simulink model "closedloop_voltage_simulation_1999v"  (R2023a)
settings: Solver=ode45  StartTime=0.0  StopTime=0.3  MaxStep=1e-4  RelTol=1e-3
settings Model: Creator=angie  LastModifiedBy=angie

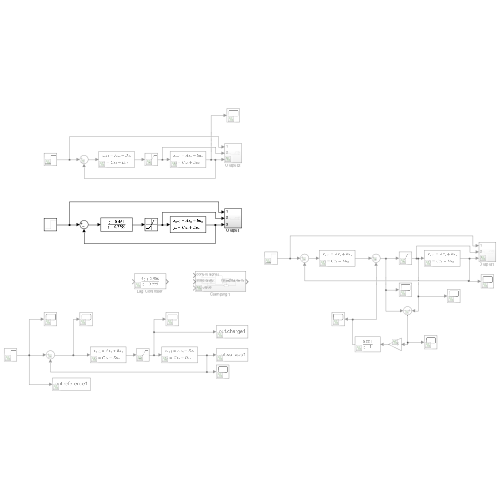
[thumbnail: Simulink's stored preview of the top-level diagram]
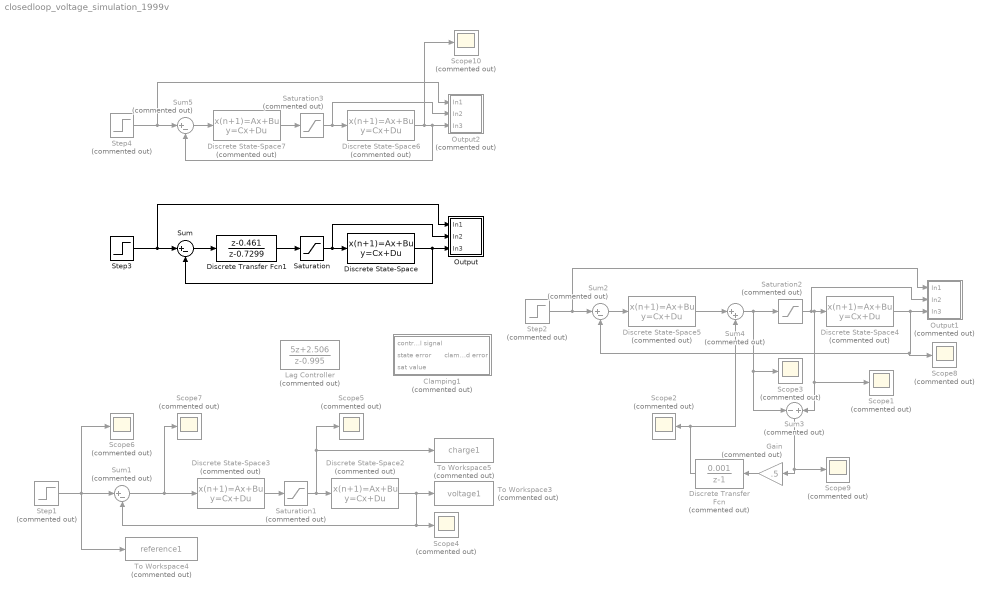
== system closedloop_voltage_simulation_1999v ==
  Clamping1 : Subsystem  Commented=on
  Discrete Transfer Fcn : DiscreteTransferFcn  Commented=on  Numerator=[0.001]  Denominator=[1 -1]  SampleTime=0.001
  Discrete Transfer Fcn1 : DiscreteTransferFcn  Numerator=[1, -0.461]  Denominator=[1 -0.7299]  SampleTime=0.001
  Discrete State-Space : DiscreteStateSpace  B=0.2728  D=0  InitialCondition=0/6  SampleTime=1/1000
  Discrete State-Space2 : DiscreteStateSpace  Commented=on  B=0.01185  D=0  InitialCondition=2000/6000  SampleTime=1/2000
  Discrete State-Space3 : DiscreteStateSpace  Commented=on  A=0.961  B=0.5099  C=0.826  D=5  SampleTime=1/2000
  Discrete State-Space4 : DiscreteStateSpace  Commented=on  B=0.0237  D=0  InitialCondition=2000/6000  SampleTime=1/1000
  Discrete State-Space5 : DiscreteStateSpace  Commented=on  A=0.9236  C=0.826  D=5  SampleTime=1/1000
  Discrete State-Space6 : DiscreteStateSpace  Commented=on  B=0.0237  D=0  InitialCondition=2/6  SampleTime=1/1000
  Discrete State-Space7 : DiscreteStateSpace  Commented=on  A=0.9236  C=0.826  D=5  SampleTime=1/1000
  Gain : Gain  Commented=on  Gain=.5
  Lag Controller : DiscreteTransferFcn  Commented=on  Numerator=[5 2.506]  Denominator=[1 -0.995]  SampleTime=1/1000
  Output : Subsystem
  Output1 : Subsystem  Commented=on
  Output2 : Subsystem  Commented=on
  Saturation : Saturate  UpperLimit=0.25  LowerLimit=-0.25
  Saturation1 : Saturate  Commented=on  UpperLimit=0.25  LowerLimit=-0.25  OutMin=-0.25  OutMax=0.25
  Saturation2 : Saturate  Commented=on  UpperLimit=0.25  LowerLimit=-0.25
  Saturation3 : Saturate  Commented=on  UpperLimit=0.25  LowerLimit=-0.25
  Scope{1..10} (10 alike) : Scope  Commented=on
  Step1 : Step  Commented=on  Before=2000/6000  After=3000/6000  SampleTime=1
  Step2 : Step  Commented=on  Time=0.1  Before=1000/6000  After=5000/6000  SampleTime=0.01
  Step3 : Step  Time=0.1  Before=0/6  After=1/6  SampleTime=0.01
  Step4 : Step  Commented=on  Time=0.1  Before=2/6  After=3/6  SampleTime=0.01
  Sum : Sum  Inputs=|+-
  Sum1 : Sum  Commented=on  Inputs=|+-
  Sum2 : Sum  Commented=on  Inputs=|+-
  Sum3 : Sum  Commented=on  Inputs=-+
  Sum4 : Sum  Commented=on  Inputs=|++
  Sum5 : Sum  Commented=on  Inputs=|+-
  To Workspace3 : ToWorkspace  Commented=on  VariableName=voltage1  SaveFormat=Timeseries  SampleTime=-1
  To Workspace4 : ToWorkspace  Commented=on  VariableName=reference1  SaveFormat=Timeseries  SampleTime=-1
  To Workspace5 : ToWorkspace  Commented=on  VariableName=charge1  SaveFormat=Timeseries  SampleTime=-1
  wires:
  Discrete State-Space/1 -> Sum/2, Output/3(In3)
  Step3/1 -> Output/1(In1), Sum/1
  Sum/1 -> Discrete Transfer Fcn1/1
  Discrete Transfer Fcn1/1 -> Saturation/1
  Saturation/1 -> Output/2(In2), Discrete State-Space/1
  Sum1/1 -> Discrete State-Space3/1, Scope7/1
  Step1/1 -> To Workspace4/1, Scope6/1, Sum1/1
  Discrete State-Space3/1 -> Saturation1/1
  Discrete State-Space2/1 -> Sum1/2, Scope4/1, To Workspace3/1
  Saturation1/1 -> To Workspace5/1, Scope5/1, Discrete State-Space2/1
  Discrete State-Space4/1 -> Scope8/1, Sum2/2, Output1/3(In3)
  Sum2/1 -> Discrete State-Space5/1
  Step2/1 -> Output1/1(In1), Sum2/1
  Gain/1 -> Discrete Transfer Fcn/1
  Discrete Transfer Fcn/1 -> Sum4/2, Scope2/1
  Saturation2/1 -> Output1/2(In2), Sum3/2, Scope1/1, Discrete State-Space4/1
  Sum3/1 -> Scope9/1, Gain/1
  Discrete State-Space5/1 -> Sum4/1
  Sum4/1 -> Scope3/1, Sum3/1, Saturation2/1
  Step4/1 -> Output2/1(In1), Sum5/1
  Saturation3/1 -> Output2/2(In2), Discrete State-Space6/1
  Discrete State-Space6/1 -> Sum5/2, Output2/3(In3), Scope10/1
  Sum5/1 -> Discrete State-Space7/1
  Discrete State-Space7/1 -> Saturation3/1

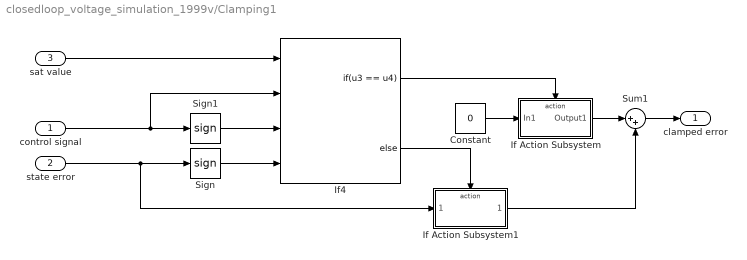
== system closedloop_voltage_simulation_1999v/Clamping1 ==
  control signal : Inport
  state error : Inport  Port=2
  sat value : Inport  Port=3
  Constant : Constant  Value=0
  If Action Subsystem : Subsystem  TreatAsAtomicUnit=on
  If Action Subsystem1 : Subsystem  TreatAsAtomicUnit=on
  If4 : If  NumInputs=4  IfExpression=u3 == u4
  Sign : Signum
  Sign1 : Signum
  Sum1 : Sum  Inputs=|++
  clamped error : Outport
  wires:
  Constant/1 -> If Action Subsystem/1(In1)
  If4/1 -> If Action Subsystem/Action
  If Action Subsystem/1(Output1) -> Sum1/1
  If Action Subsystem1/1(Output2) -> Sum1/2
  If4/2 -> If Action Subsystem1/Action
  control signal/1 -> If4/2, Sign1/1
  sat value/1 -> If4/1
  Sum1/1 -> clamped error/1
  Sign1/1 -> If4/3
  Sign/1 -> If4/4
  state error/1 -> If Action Subsystem1/1(state error), Sign/1

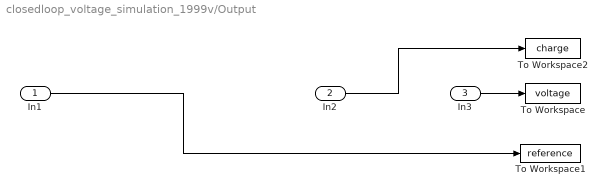
== system closedloop_voltage_simulation_1999v/Output ==
  In1 : Inport
  In2 : Inport  Port=2
  In3 : Inport  Port=3
  To Workspace : ToWorkspace  VariableName=voltage  SaveFormat=Timeseries  SampleTime=-1
  To Workspace1 : ToWorkspace  VariableName=reference  SaveFormat=Timeseries  SampleTime=-1
  To Workspace2 : ToWorkspace  VariableName=charge  SaveFormat=Timeseries  SampleTime=-1
  wires:
  In3/1 -> To Workspace/1
  In2/1 -> To Workspace2/1
  In1/1 -> To Workspace1/1

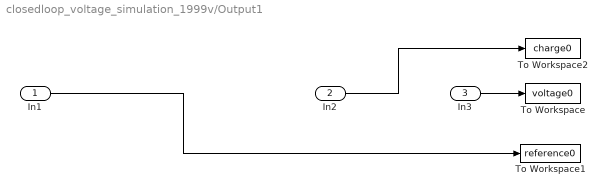
== system closedloop_voltage_simulation_1999v/Output1 ==
  In1 : Inport
  In2 : Inport  Port=2
  In3 : Inport  Port=3
  To Workspace : ToWorkspace  VariableName=voltage0  SaveFormat=Timeseries  SampleTime=-1
  To Workspace1 : ToWorkspace  VariableName=reference0  SaveFormat=Timeseries  SampleTime=-1
  To Workspace2 : ToWorkspace  VariableName=charge0  SaveFormat=Timeseries  SampleTime=-1
  wires:
  In3/1 -> To Workspace/1
  In2/1 -> To Workspace2/1
  In1/1 -> To Workspace1/1

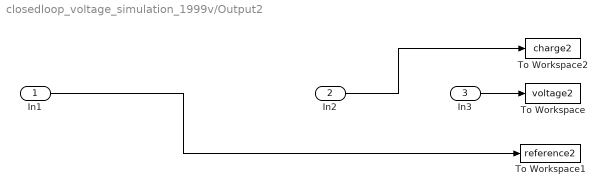
== system closedloop_voltage_simulation_1999v/Output2 ==
  In1 : Inport
  In2 : Inport  Port=2
  In3 : Inport  Port=3
  To Workspace : ToWorkspace  VariableName=voltage2  SaveFormat=Timeseries  SampleTime=-1
  To Workspace1 : ToWorkspace  VariableName=reference2  SaveFormat=Timeseries  SampleTime=-1
  To Workspace2 : ToWorkspace  VariableName=charge2  SaveFormat=Timeseries  SampleTime=-1
  wires:
  In3/1 -> To Workspace/1
  In2/1 -> To Workspace2/1
  In1/1 -> To Workspace1/1

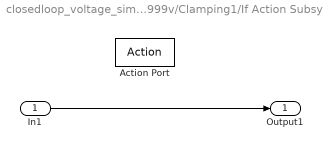
== system closedloop_voltage_simulation_1999v/Clamping1/If Action Subsystem ==
  In1 : Inport
  Action Port : ActionPort  ActionPortLabel=if(u3 == u4)
  Output1 : Outport
  wires:
  In1/1 -> Output1/1

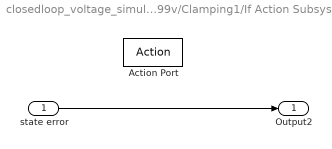
== system closedloop_voltage_simulation_1999v/Clamping1/If Action Subsystem1 ==
  state error : Inport
  Action Port : ActionPort  ActionPortLabel=else
  Output2 : Outport
  wires:
  state error/1 -> Output2/1
